simulink subsystem "INIT"  (R2023b)
settings: Solver=VariableStepAuto  StartTime=0.0  StopTime=10.0  RelTol=1e-3
libraries: simulink x1
settings Model: Creator=diego  LastModifiedBy=rebek

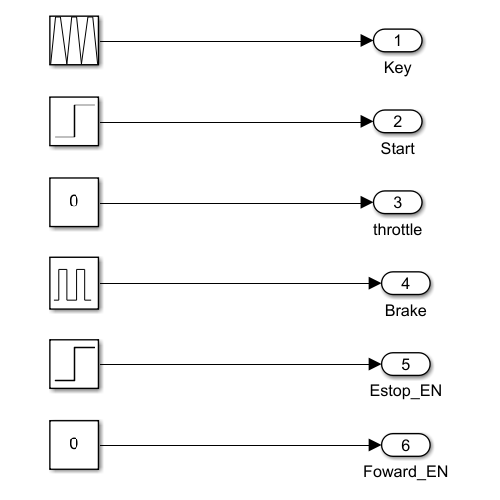
[thumbnail: Simulink's stored preview of the top-level diagram]
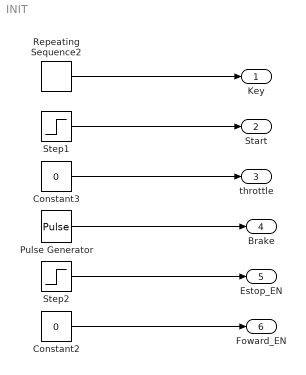
== system INIT ==
  Constant2 : Constant  Value=0
  Constant3 : Constant  Value=0
  Pulse Generator : DiscretePulseGenerator  PulseType=Time based  Period=100  PulseWidth=50
  Repeating Sequence2 : simulink/Sources/Repeating Sequence  rep_seq_t=[0 100 200 300]  rep_seq_y=[0 1 1 0]
  Step1 : Step  Time=200  SampleTime=0
  Step2 : Step  Time=400  SampleTime=0
  Key : Outport
  Start : Outport  Port=2
  throttle : Outport  Port=3
  Brake : Outport  Port=4
  Estop_EN : Outport  Port=5
  Foward_EN : Outport  Port=6
  wires:
  Constant3/1 -> throttle/1
  Pulse Generator/1 -> Brake/1
  Step1/1 -> Start/1
  Repeating Sequence2/1 -> Key/1
  Step2/1 -> Estop_EN/1
  Constant2/1 -> Foward_EN/1
